simulink model "panel_AS6"  (R2018a)
settings: Solver=VariableStepAuto  StartTime=0.0  StopTime=10.0  RelTol=1e-3  EnableMultiTasking=on
undefined symbols (not defined in the file): Eg0, Gn, Isc, K, Ki, n, Ns, q, Rp, Rs, Tn, Voc
libraries: simulink x3
settings Model: Creator=PC  LastModifiedBy=yassine
settings OptimizationCC: LifeSpan=inf
settings DebuggingCC: SFUnexpectedBacktrackingDiag=warning  SFNoUnconditionalDefaultTransitionDiag=warning
settings CodeAppCC: StateflowObjectComments=on
settings GRTTargetCC: TargetLangStandard=C89/C90 (ANSI)
settings ConfigComp: CovMetricSettings=dw  CovSaveCumulativeToWorkspaceVar=on  CovSaveSingleToWorkspaceVar=on  CovExternalEMLEnable=off

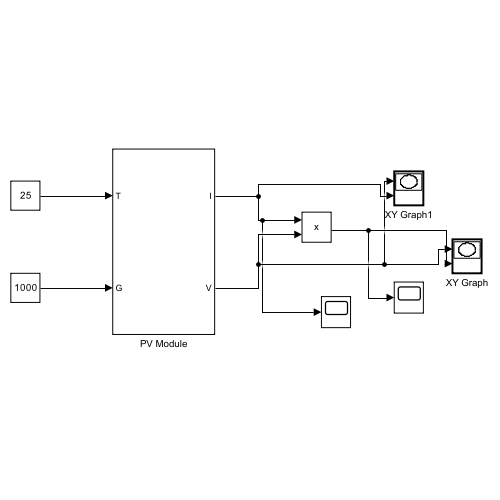
[thumbnail: Simulink's stored preview of the top-level diagram]
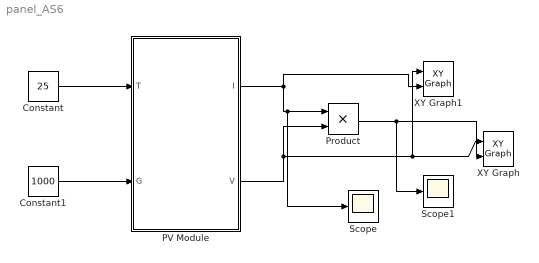
== system panel_AS6 ==
  Constant : Constant  Value=25
  Constant1 : Constant  Value=1000
  PV Module : Subsystem  InitFcn=|
      | Ki=5e-4;
      | q=1.6e-19;
      | K=1.38e-23;
      | n=1.3;
      | Eg0=1.12;
      | Rs=.1;
      | Rp=515;
      | Tn=298.15;
      | Gn=1000;
      | Voc=46.5;
      | Isc=9.68;
      | Ns=72;
  Product : Product
  Scope : Scope
  Scope1 : Scope
  XY Graph : simulink/Sinks/XY Graph  xmin=-1  xmax=1  ymin=-1  ymax=1  st=-1
  XY Graph1 : simulink/Sinks/XY Graph  xmin=-1  xmax=1  ymin=-1  ymax=1  st=-1
  wires:
  Constant1/1 -> PV Module/2(G)
  Constant/1 -> PV Module/1(T)
  PV Module/1(I) -> XY Graph1/2, Scope/1, Product/1
  PV Module/2(V) -> XY Graph/1, XY Graph1/1, Product/2
  Product/1 -> Scope1/1, XY Graph/2

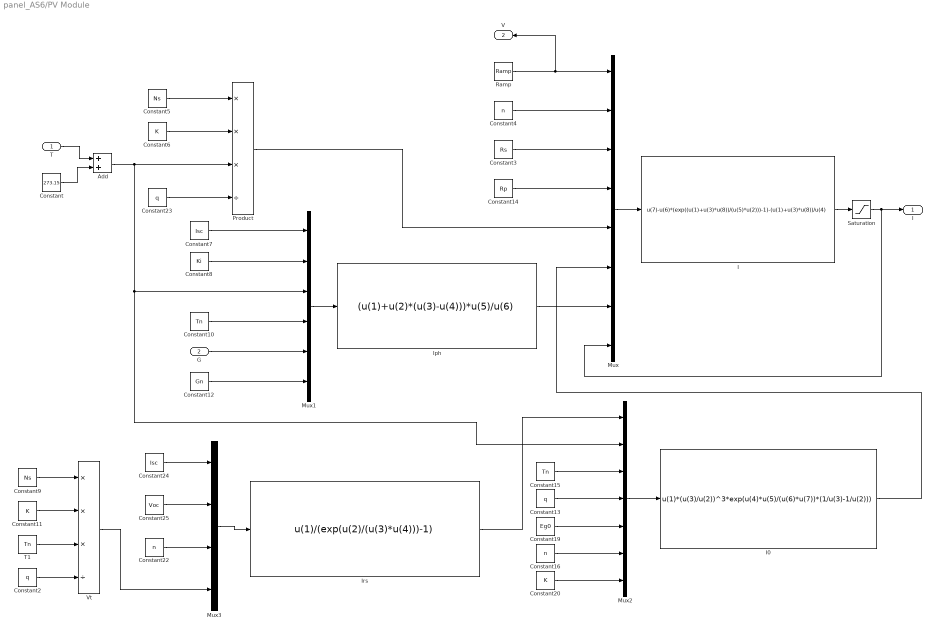
== system panel_AS6/PV Module ==
  T : Inport
  G : Inport  Port=2
  Add : Sum
  Constant : Constant  Value=273.15
  Constant10 : Constant  Value=Tn
  Constant11 : Constant  Value=K
  Constant12 : Constant  Value=Gn
  Constant13 : Constant  Value=q
  Constant14 : Constant  Value=Rp
  Constant15 : Constant  Value=Tn
  Constant16 : Constant  Value=n
  Constant19 : Constant  Value=Eg0
  Constant2 : Constant  Value=q
  Constant20 : Constant  Value=K
  Constant22 : Constant  Value=n
  Constant23 : Constant  Value=q
  Constant24 : Constant  Value=Isc
  Constant25 : Constant  Value=Voc
  Constant3 : Constant  Value=Rs
  Constant4 : Constant  Value=n
  Constant5 : Constant  Value=Ns
  Constant6 : Constant  Value=K
  Constant7 : Constant  Value=Isc
  Constant8 : Constant  Value=Ki
  Constant9 : Constant  Value=Ns
  "I " : Fcn  Expr=u(7)-u(6)*(exp((u(1)+u(3)*u(8))/(u(5)*u(2)))-1)-(u(1)+u(3)*u(8))/u(4)
  I0 : Fcn  Expr=u(1)*(u(3)/u(2))^3*exp(u(4)*u(5)/(u(6)*u(7))*(1/u(3)-1/u(2)))
  Iph : Fcn  Expr=(u(1)+u(2)*(u(3)-u(4)))*u(5)/u(6)
  Irs : Fcn  Expr=u(1)/(exp(u(2)/(u(3)*u(4)))-1)
  Mux : Mux  Inputs=8
  Mux1 : Mux  Inputs=6
  Mux2 : Mux  Inputs=7
  Mux3 : Mux
  Product : Product  Inputs=***/
  Ramp : simulink/Sources/Ramp  slope=6  start=0  InitialOutput=0
  Saturation : Saturate  UpperLimit=10  LowerLimit=0
  T1 : Constant  Value=Tn
  Vt : Product  Inputs=***/
  I : Outport
  V : Outport  Port=2
  wires:
  Constant5/1 -> Product/1
  Constant20/1 -> Mux2/7
  Constant4/1 -> Mux/2
  Constant3/1 -> Mux/3
  Product/1 -> Mux/5
  Ramp/1 -> V/1, Mux/1
  Mux/1 -> "I "/1
  Constant14/1 -> Mux/4
  Mux1/1 -> Iph/1
  Constant8/1 -> Mux1/2
  Constant10/1 -> Mux1/4
  G/1 -> Mux1/5
  Iph/1 -> Mux/7
  Constant7/1 -> Mux1/1
  Constant12/1 -> Mux1/6
  Constant15/1 -> Mux2/3
  Mux2/1 -> I0/1
  Constant13/1 -> Mux2/4
  Constant19/1 -> Mux2/5
  I0/1 -> Mux/6
  Constant16/1 -> Mux2/6
  Add/1 -> Mux2/2, Mux1/3, Product/3
  Mux3/1 -> Irs/1
  Constant24/1 -> Mux3/1
  Constant22/1 -> Mux3/3
  Constant25/1 -> Mux3/2
  Irs/1 -> Mux2/1
  Constant2/1 -> Vt/4
  T1/1 -> Vt/3
  Constant9/1 -> Vt/1
  Constant11/1 -> Vt/2
  Vt/1 -> Mux3/4
  Constant6/1 -> Product/2
  Constant23/1 -> Product/4
  "I "/1 -> Saturation/1
  Constant/1 -> Add/2
  T/1 -> Add/1
  Saturation/1 -> I/1, Mux/8
